simulink model "ControladorAtuadorHidraulico"  (R2015a)
settings: Solver=ode45  StartTime=0.0  StopTime=10  FixedStep=1  RelTol=1e-3
settings Model: Creator=Wagner  LastModifiedBy=Wagner
settings SolverCC: ZeroCrossAlgorithm=Adaptive
settings DataIOCC: LimitDataPoints=off

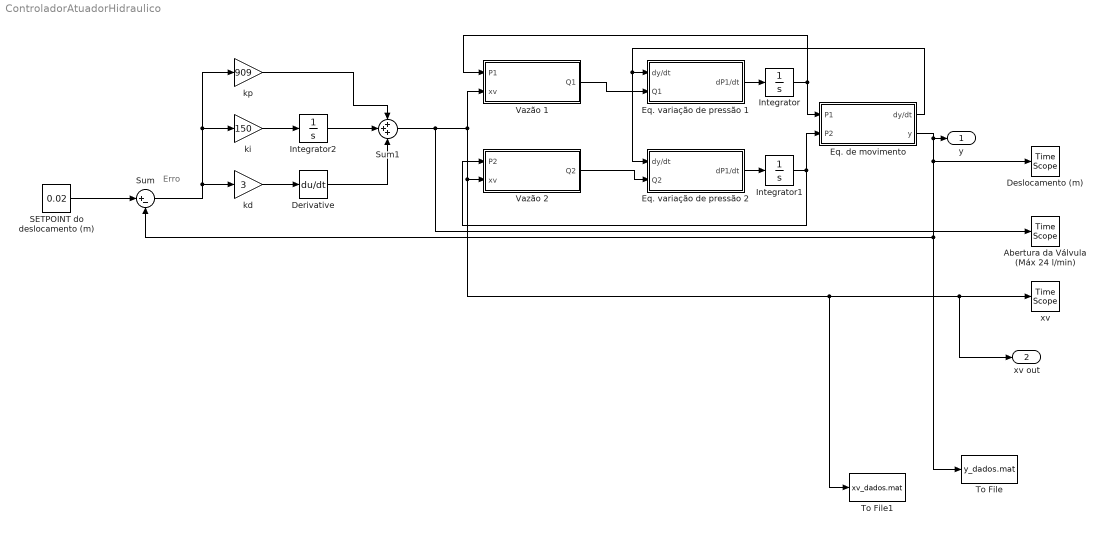
== system ControladorAtuadorHidraulico ==
  note: Erro
  Abertura da Válvula (Máx 24 l/min) : TimeScope
  Derivative : Derivative
  Deslocamento (m) : TimeScope
  Eq. de movimento : Subsystem
  Eq. variação de pressão 1 : Subsystem
  Eq. variação de pressão 2 : Subsystem
  Integrator : Integrator
  Integrator1 : Integrator
  Integrator2 : Integrator
  SETPOINT do deslocamento (m) : Constant  Value=0.02
  Sum : Sum  Inputs=|+-
  Sum1 : Sum  Inputs=+++
  To File : ToFile  Filename=y_dados.mat  MatrixName=y
  To File1 : ToFile  Filename=xv_dados.mat  MatrixName=xv
  Vazão 1 : Subsystem
  Vazão 2 : Subsystem
  kd : Gain  Gain=3
  ki : Gain  Gain=150
  kp : Gain  Gain=909
  xv : TimeScope
  y : Outport
  xv out : Outport  Port=2
  wires:
  Vazão 2/1(Q2) -> Eq. variação de pressão 2/2(Q2)
  Eq. variação de pressão 1/1(dP1/dt) -> Integrator/1
  Eq. variação de pressão 2/1(dP1/dt) -> Integrator1/1
  Integrator1/1 -> Vazão 2/1(P2), Eq. de movimento/2(P2)
  Integrator/1 -> Eq. de movimento/1(P1), Vazão 1/1(P1)
  Eq. de movimento/1(dy/dt) -> Eq. variação de pressão 1/1(dy/dt), Eq. variação de pressão 2/1(dy/dt)
  Vazão 1/1(Q1) -> Eq. variação de pressão 1/2(Q1)
  Eq. de movimento/2(y) -> To File/1, Sum/2, Deslocamento (m)/1, y/1
  Sum1/1 -> Vazão 1/2(xv), To File1/1, xv out/1, xv/1, Vazão 2/2(xv), Abertura da Válvula (Máx 24 l/min)/1
  Sum/1 -> kp/1, ki/1, kd/1
  ki/1 -> Integrator2/1
  kd/1 -> Derivative/1
  kp/1 -> Sum1/1
  Integrator2/1 -> Sum1/2
  Derivative/1 -> Sum1/3
  SETPOINT do deslocamento (m)/1 -> Sum/1

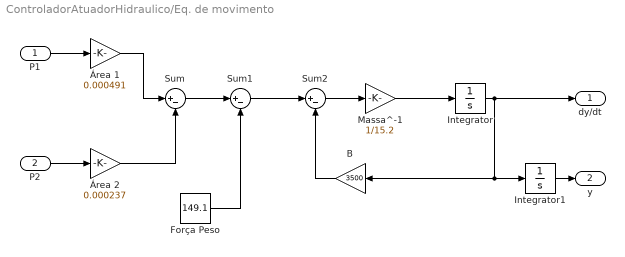
== system ControladorAtuadorHidraulico/Eq. de movimento ==
  P1 : Inport
  P2 : Inport  Port=2
  B : Gain  Gain=3500
  Força Peso : Constant  Value=149.1
  Integrator : Integrator
  Integrator1 : Integrator
  Massa^-1 : Gain  Gain=1/15.2
  Sum : Sum  Inputs=|+-
  Sum1 : Sum  Inputs=|+-
  Sum2 : Sum  Inputs=|+-
  Área 1 : Gain  Gain=0.000491
  Área 2 : Gain  Gain=0.000237
  dy/dt : Outport
  y : Outport  Port=2
  wires:
  P1/1 -> Área 1/1
  Área 1/1 -> Sum/1
  P2/1 -> Área 2/1
  Área 2/1 -> Sum/2
  Sum/1 -> Sum1/1
  Sum1/1 -> Sum2/1
  Sum2/1 -> Massa^-1/1
  Massa^-1/1 -> Integrator/1
  B/1 -> Sum2/2
  Integrator/1 -> B/1, Integrator1/1, dy/dt/1
  Integrator1/1 -> y/1
  Força Peso/1 -> Sum1/2

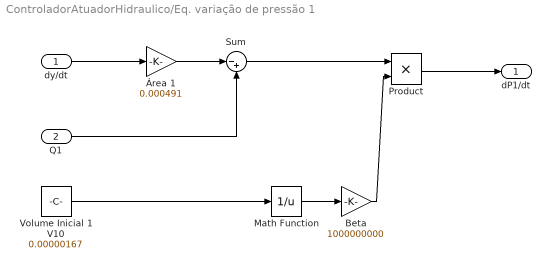
== system ControladorAtuadorHidraulico/Eq. variação de pressão 1 ==
  dy/dt : Inport
  Q1 : Inport  Port=2
  Beta : Gain  Gain=1000000000
  Math Function : Math  Operator=reciprocal  RndMeth=Zero  SaturateOnIntegerOverflow=on
  Product : Product
  Sum : Sum  Inputs=|-+
  Volume Inicial 1 V10 : Constant  Value=0.00000167
  Área 1 : Gain  Gain=0.000491
  dP1/dt : Outport
  wires:
  dy/dt/1 -> Área 1/1
  Área 1/1 -> Sum/1
  Q1/1 -> Sum/2
  Sum/1 -> Product/1
  Beta/1 -> Product/2
  Math Function/1 -> Beta/1
  Product/1 -> dP1/dt/1
  Volume Inicial 1 V10/1 -> Math Function/1

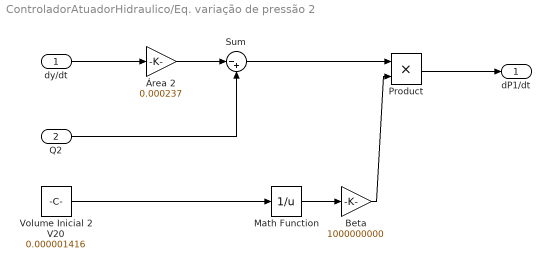
== system ControladorAtuadorHidraulico/Eq. variação de pressão 2 ==
  dy/dt : Inport
  Q2 : Inport  Port=2
  Beta : Gain  Gain=1000000000
  Math Function : Math  Operator=reciprocal  RndMeth=Zero  SaturateOnIntegerOverflow=on
  Product : Product
  Sum : Sum  Inputs=|-+
  Volume Inicial 2 V20 : Constant  Value=0.000001416
  Área 2 : Gain  Gain=0.000237
  dP1/dt : Outport
  wires:
  dy/dt/1 -> Área 2/1
  Área 2/1 -> Sum/1
  Q2/1 -> Sum/2
  Sum/1 -> Product/1
  Beta/1 -> Product/2
  Math Function/1 -> Beta/1
  Product/1 -> dP1/dt/1
  Volume Inicial 2 V20/1 -> Math Function/1

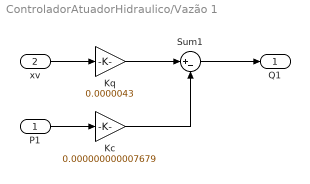
== system ControladorAtuadorHidraulico/Vazão 1 ==
  P1 : Inport
  xv : Inport  Port=2
  Kc : Gain  Gain=0.000000000007679
  Kq : Gain  Gain=0.0000043
  Sum1 : Sum  Inputs=|+-
  Q1 : Outport
  wires:
  Kq/1 -> Sum1/1
  Sum1/1 -> Q1/1
  xv/1 -> Kq/1
  P1/1 -> Kc/1
  Kc/1 -> Sum1/2

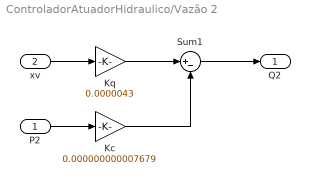
== system ControladorAtuadorHidraulico/Vazão 2 ==
  P2 : Inport
  xv : Inport  Port=2
  Kc : Gain  Gain=0.000000000007679
  Kq : Gain  Gain=0.0000043
  Sum1 : Sum  Inputs=|+-
  Q2 : Outport
  wires:
  Kq/1 -> Sum1/1
  Sum1/1 -> Q2/1
  xv/1 -> Kq/1
  P2/1 -> Kc/1
  Kc/1 -> Sum1/2
